simulink model "Simulink_2369656"  (R2025b)
settings: Solver=VariableStepAuto  StartTime=0.0  StopTime=10.0  RelTol=1e-3
settings Model: Creator=elias  LastModifiedBy=elias

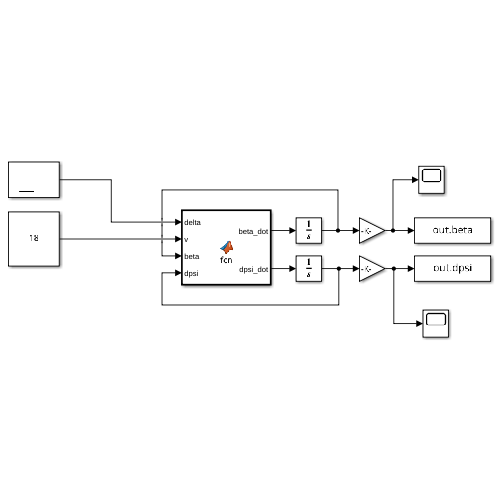
[thumbnail: Simulink's stored preview of the top-level diagram]
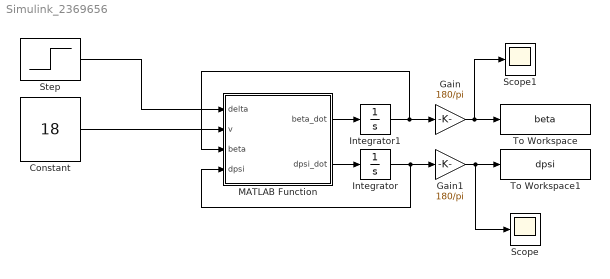
== system Simulink_2369656 ==
  Constant : Constant  Value=18
  Gain : Gain  Gain=180/pi
  Gain1 : Gain  Gain=180/pi
  Integrator : Integrator
  Integrator1 : Integrator
  MATLAB Function : MATLAB Function  TreatAsAtomicUnit=on
  Scope : Scope
      settings: ActiveDisplayYMinimum=-1  ActiveDisplayYMaximum=1
  Scope1 : Scope
      settings: ActiveDisplayYMinimum=-1.0539462341281665  ActiveDisplayYMaximum=0.55971155965507424
  Step : Step  Time=0  After=5 * pi / 180  SampleTime=0
  To Workspace : ToWorkspace  VariableName=beta  SaveFormat=Timeseries  SampleTime=-1
  To Workspace1 : ToWorkspace  VariableName=dpsi  SaveFormat=Timeseries  SampleTime=-1
  wires:
  Step/1 -> MATLAB Function/1(delta)
  Constant/1 -> MATLAB Function/2(v)
  MATLAB Function/2(dpsi_dot) -> Integrator/1
  MATLAB Function/1(beta_dot) -> Integrator1/1
  Integrator1/1 -> Gain/1, MATLAB Function/3(beta)
  Integrator/1 -> Gain1/1, MATLAB Function/4(dpsi)
  Gain/1 -> Scope1/1, To Workspace/1
  Gain1/1 -> Scope/1, To Workspace1/1

== matlab function Simulink_2369656/MATLAB Function ==
  data: delta input; beta_dot output; v input; beta input; dpsi input; dpsi_dot output; p parameter
function [beta_dot, dpsi_dot] = fcn(delta, v, beta, dpsi, p)

cb = cos(beta);

% 1. Schräglaufwinkel berechnen (mit Parametern aus dem Struct p)
    alpha_v = delta - (p.lf * dpsi) / (v * cb) + tan(beta);
    alpha_h = (p.lr * dpsi) / (v * cb) - tan(beta);

    % Reifen-Seitenkräfte (wie in deinem Skript)
    Fy_v = p.cf * alpha_v;
    Fy_h = p.cr * alpha_h;

    % 2. Differentialgleichungen (Zustandsableitungen)
    beta_dot = -dpsi + (1 / (p.m * v)) * ((Fy_v * cos(delta) / cb) + (Fy_h / cb));
    dpsi_dot = (1 / p.Jz) * (p.lf * Fy_v * cos(delta) - p.lr * Fy_h);

end
